simulink model "matlab_advance_MPC_opc_opre"  (R2018b)
settings: Solver=VariableStepAuto  StartTime=0.0  StopTime=40  RelTol=1e-3
undefined symbols (not defined in the file or in its folder): AI1, AO1, Dev1
libraries: opclib x3, mpclib x1
settings Model: Creator=erange  LastModifiedBy=erange

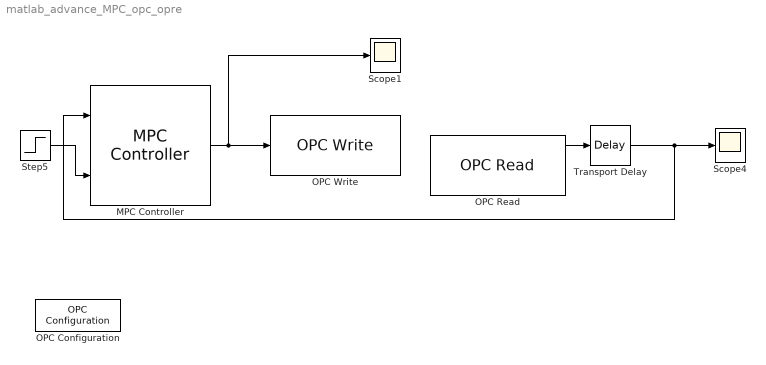
== system matlab_advance_MPC_opc_opre ==
  MPC Controller : mpclib/MPC Controller  SCDEnableBlockLinearizationSpecification=on  mpcobj=mpc2  is_multiple=0  enable_value=0  return_u0=off  updateMPCinCallerWorkspace=on  md_inport=off  mv_inport=off  return_cost=off  return_mvseq=off  return_qpstatus=off  return_xseq=off  return_state=off  return_ovseq=off  state_inport=off  umin_inport=off  umax_inport=off  ymin_inport=off  ymax_inport=off  cc_inport=off  ywt_inport=off  uwt_inport=off  duwt_inport=off  rhoeps_inport=off  uref_inport=off  n_ts=0.01  n_p=500  n_mv=1  n_md=0  n_ud=0  n_mo=1  n_uo=0  BlockDataType=double  SampleTimeInherited=off  switch_inport=off
  OPC Configuration : opclib/OPC Configuration  opcServers=localhost/NI USB-6008.Server/10, localhost/Tank2.Server/10  errMissingItems=Error  errReadWrite=Warn  errShutdown=Error  errRTViolation=Warn  rtEnable=on  speedup=1  showLatency=off  beingUsed=on
      settings: SourceProductName=OPC Toolbox  SourceProductBaseCode=OT
  OPC Read : opclib/OPC Read  serverHost=localhost  serverID=NI USB-6008.Server  itemIDs=Dev1/AI1  readMode=Synchronous (cache)  dataType=double  updateRate=0.01  showQual=on  showTS=on  tsMode=Seconds since start
      settings: SourceProductName=OPC Toolbox  SourceProductBaseCode=OT
  OPC Write : opclib/OPC Write  serverHost=localhost  serverID=NI USB-6008.Server  itemIDs=Dev1/AO1  writeMode=Synchronous  updateRate=0
      settings: SourceProductName=OPC Toolbox  SourceProductBaseCode=OT
  Scope1 : Scope
  Scope4 : Scope
  Step5 : Step  Time=0  SampleTime=1
  Transport Delay : TransportDelay  DelayTime=3
  wires:
  Step5/1 -> MPC Controller/2
  MPC Controller/1 -> OPC Write/1, Scope1/1
  OPC Read/1 -> Transport Delay/1
  Transport Delay/1 -> MPC Controller/1, Scope4/1
